simulink model "SCIM01"  (R2016a)
settings: Solver=FixedStepAuto  StartTime=0.0  StopTime=1  FixedStep=0.0001  RelTol=1e-3
values from neighbouring files (symbols this model uses):
  A = [1  2  3; 4  5  6]    [motor4_workspace.mat]    (also in stationary.m = [A11,  om_coord,  A13,  A14; stationary_class.m = []; torqueFinder.m = [A11,  om_coord,  A13,  A14; workspaceSav.mat = [-369.480519481 0 3.90909090909 0 0 -369.480519481 0 3.90909)
  B = [1/Ls/sig, 0 ... (first row only)    [stationary.m]    (also in stationary_class.m = []; torqueFinder.m; workspaceSav.mat = [52.380952381  0; 0  52.380952381; 0  0; 0  0])
  Lm = 0.1271    [motor4_workspace.mat]    (also in motor_wrapper.m = obj.Lm; scim_verifier.m = obj.motor.getLm(); setMotorParams.m; stationary_class.m = obj.Lm)
  Lr = 0.2744    [motor4_workspace.mat]    (also in motor_wrapper.m = obj.Lr; scim_verifier.m = obj.motor.getLr(); setMotorParams.m; stationary_class.m = obj.Lr)
settings Model: Creator=ebenera  LastModifiedBy=ebenera

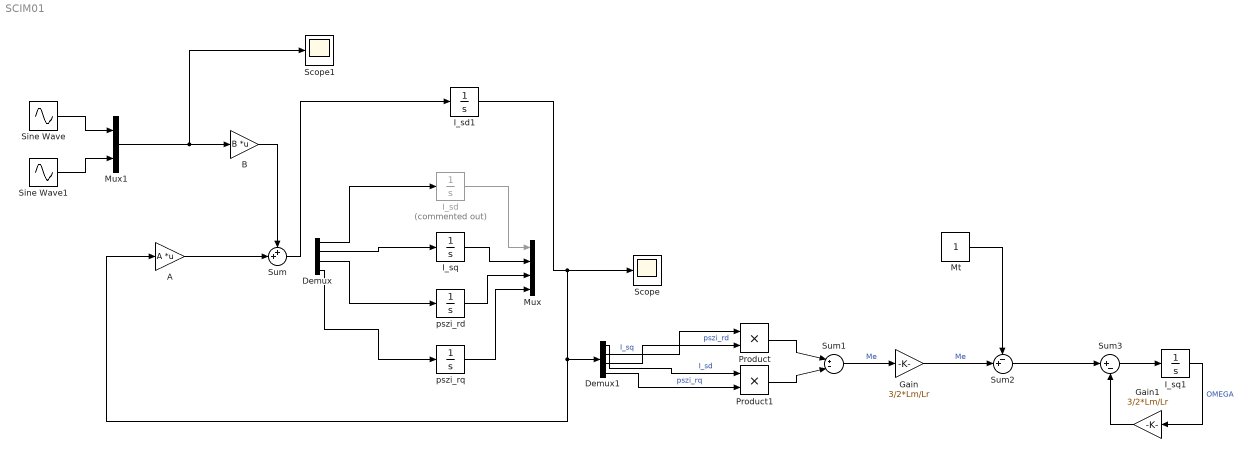
== system SCIM01 ==
  A : Gain  Gain=A  Multiplication=Matrix(K*u)
  B : Gain  Gain=B  Multiplication=Matrix(K*u)
  Demux : Demux
  Demux1 : Demux
  Gain : Gain  Gain=3/2*Lm/Lr
  Gain1 : Gain  Gain=3/2*Lm/Lr
  I_sd : Integrator  Commented=on  ContinuousStateAttributes='i_sd'
  I_sd1 : Integrator  ContinuousStateAttributes='i_sd'
  I_sq : Integrator
  I_sq1 : Integrator
  Mt : Constant
  Mux : Mux
  Mux1 : Mux  Inputs=2
  Product : Product
  Product1 : Product
  Scope : Scope
  Scope1 : Scope
  Sine Wave : Sin  Amplitude=0.8  Frequency=314  SampleTime=0
  Sine Wave1 : Sin  Amplitude=0.8  Frequency=314  Phase=1.5  SampleTime=0
  Sum : Sum  Inputs=++|
  Sum1 : Sum  Inputs=|+-|
  Sum2 : Sum  Inputs=-+|
  Sum3 : Sum  Inputs=|+-
  pszi_rd : Integrator
  "pszi_rq " : Integrator
  wires:
  I_sd/1 -> Mux/1
  I_sq/1 -> Mux/2
  pszi_rd/1 -> Mux/3
  "pszi_rq "/1 -> Mux/4
  I_sd1/1 -> Scope/1, Demux1/1, A/1
  Demux/1 -> I_sd/1
  Demux/4 -> "pszi_rq "/1
  Demux/3 -> pszi_rd/1
  Demux/2 -> I_sq/1
  Sum/1 -> I_sd1/1
  A/1 -> Sum/2
  B/1 -> Sum/1
  Mux1/1 -> Scope1/1, B/1
  Sine Wave1/1 -> Mux1/2
  Sine Wave/1 -> Mux1/1
  Demux1/1 -> Product1/1  "I_sd"
  Demux1/2 -> Product/1  "I_sq"
  Demux1/3 -> Product/2  "pszi_rd"
  Demux1/4 -> Product1/2  "pszi_rq"
  Product/1 -> Sum1/1
  Product1/1 -> Sum1/2
  Sum1/1 -> Gain/1  "Me"
  Gain/1 -> Sum2/2  "Me"
  Mt/1 -> Sum2/1
  Sum2/1 -> Sum3/1
  Gain1/1 -> Sum3/2
  Sum3/1 -> I_sq1/1
  I_sq1/1 -> Gain1/1  "OMEGA"
